simulink model "cst_robotarm1"  (R2020a)
settings: Solver=ode23t  StartTime=0.0  StopTime=5  FixedStep=0.0001  MaxStep=0.05  RelTol=1e-3  EnableMultiTasking=on
model workspace (MAT data in the model file):
  DCMotor_J = 0.0946866703633
  DCMotor_K = 0.477771340295
  DCMotor_Kf = 0.921434142151
  DCMotor_L = 0.000316454712175
  DCMotor_R = 4.99938152603
  Ts = 0.1
  dFilt = [1 -0.1202]
  nFilt = [0.4399 0.4399]
undefined symbols (not defined in the file or in its folder): X, Y, Z
libraries: sm_lib x244, fl_lib x75, nesl_utility x28, ee_lib x21, simulink x6
(part 1 of 6)
settings Model: SimulationMode=accelerator  Creator=The MathWorks, Inc.  LastModifiedBy=nikhil
settings DataIOCC: LimitDataPoints=on  SaveFormat=Array  InspectSignalLogs=on  SaveTime=off  ReturnWorkspaceOutputs=off
settings OptimizationCC: ExpressionDepthLimit=2147483647  LifeSpan=inf
settings DebuggingCC: UnderspecifiedInitializationDetection=Classic  MergeDetectMultiDrivingBlocksExec=none  FcnCallInpInsideContextMsg=warning  StateNameClashWarn=warning  SFUnexpectedBacktrackingDiag=warning  SFNoUnconditionalDefaultTransitionDiag=warning  SFExecutionAtInitializationDiag=none  ArithmeticOperatorsInVariantConditions=warning
settings HardwareCC: ProdBitPerPointer=32  ProdBitPerSizeT=32  ProdBitPerPtrDiffT=32  ProdLargestAtomicFloat=None  ProdIntDivRoundTo=Undefined  ProdEndianess=Unspecified  ProdWordSize=32  ProdHWDeviceType=32-bit Generic
settings ModelReferenceCC: PropagateSignalLabelsOutOfModel=off
settings SFSimCC: SimUseLocalCustomCode=off  CustomCodeUndefinedFunction=UseInterfaceOnly
settings RTWCC: RTWUseLocalCustomCode=off
settings CodeAppCC: StateflowObjectComments=on
settings GRTTargetCC: TargetLangStandard=C89/C90 (ANSI)  CombineOutputUpdateFcns=off  GRTInterface=on
settings ConfigComp: CovMetricSettings=dw  CovHtmlReporting=on  CovSaveCumulativeToWorkspaceVar=on  CovSaveSingleToWorkspaceVar=on  CovExternalEMLEnable=off  CovSFcnEnable=off
settings SimscapeCC: SimscapeNormalizeSystem=off
settings ConfigurationSet: Description=SimMechanics 2G
settings DiagnosticsConfigSet: SimMechanicsUnconnectedFramePorts=none
settings ExplorerConfigSet: SimMechanicsOpenEditorOnUpdate=off  InternalSimMechanicsExplorerSettings="<ExplorerConfiguration><canonicalview>planar_xy</canonicalview><AnimationSetting><BasePlaybackSpeed>1.0</BasePlaybackSpeed><PlaybackSpeedFactor>1.0</PlaybackSpeedFactor></AnimationSetting><TilePanel><TileInfo><Tiles Columns=\"1\" Count=\"1\" Rows=\"1\"><Column Left=\"2\" Weight=\"1\"/><Column Left=\"708\"/><Row Top=\"2\" Weight=\"1\"/><Row Top=\"595\"/><Tile Height=\"1\" Width=\"1\" X=\"0\" Y=\"0\"/></Tiles></TileInfo><SceneInfo><SceneViewer><BGColor><R>0.80000001192092896</R><G>0.80000001192092896</G><B>0.80000001192092896</B></BGColor><Camera><Position><X>0.30752487944302698</X><Y>0.57922836563106395</Y><Z>0.35651305744246536</Z></Position><Center><X>-0.033772386749033274</X><Y>0.23793109943898419</Y><Z>0.015215791250393121</Z></Center><Up><X>-0.40824829046386307</X><Y>0.81649658092772615</Y><Z>-0.40824829046386307</Z></Up><Left>-0.063283674940751766</Left><Right>0.063283674940751766</Right><Bottom>-0.22321517040744418</Bottom><Top>0.22321517040744418</Top></Camera></SceneViewer></SceneInfo></TilePanel></ExplorerConfiguration>"

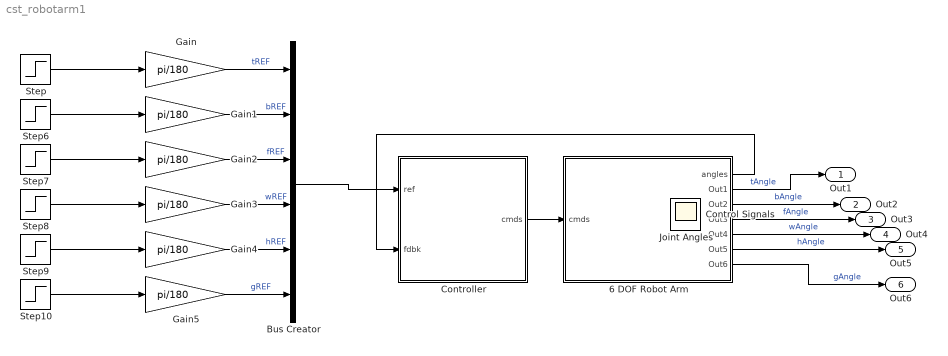
== system cst_robotarm1 ==
  6 DOF Robot Arm : Subsystem
      mask Display: image('RobotArmSystem.jpg',[0.2 0.05 0.6 0.9])
  Bus Creator : BusCreator  Inputs=6
  Controller : Subsystem
  Gain{,1..5} (6 alike) : Gain  Gain=pi/180
  Step : Step  Time=0  After=60  SampleTime=Ts
  Step10 : Step  Time=0  After=60  SampleTime=Ts
  Step6 : Step  Time=0  Before=90  After=80  SampleTime=Ts
  Step7 : Step  Time=0  After=60  SampleTime=Ts
  Step8 : Step  Time=0  After=90  SampleTime=Ts
  Step9 : Step  Time=0  After=90  SampleTime=Ts
  Out1 : Outport
  Out2 : Outport  Port=2
  Out3 : Outport  Port=3
  Out4 : Outport  Port=4
  Out5 : Outport  Port=5
  Out6 : Outport  Port=6
  Control Signals : Scope
  Joint Angles : Scope
  wires:
  Controller/1(cmds) -> 6 DOF Robot Arm/1(cmds)
  6 DOF Robot Arm/1(angles) -> Controller/2(fdbk)
  Gain4/1 -> Bus Creator/5  "hREF"
  Gain/1 -> Bus Creator/1  "tREF"
  Gain3/1 -> Bus Creator/4  "wREF"
  Gain5/1 -> Bus Creator/6  "gREF"
  Gain1/1 -> Bus Creator/2  "bREF"
  Step9/1 -> Gain4/1
  Step/1 -> Gain/1
  Step10/1 -> Gain5/1
  Bus Creator/1 -> Controller/1(ref)
  Gain2/1 -> Bus Creator/3  "fREF"
  Step7/1 -> Gain2/1
  Step8/1 -> Gain3/1
  Step6/1 -> Gain1/1
  6 DOF Robot Arm/2(Out1) -> Out1/1  "tAngle"
  6 DOF Robot Arm/3(Out2) -> Out2/1  "bAngle"
  6 DOF Robot Arm/4(Out3) -> Out3/1  "fAngle"
  6 DOF Robot Arm/5(Out4) -> Out4/1  "wAngle"
  6 DOF Robot Arm/6(Out5) -> Out5/1  "hAngle"
  6 DOF Robot Arm/7(Out6) -> Out6/1  "gAngle"

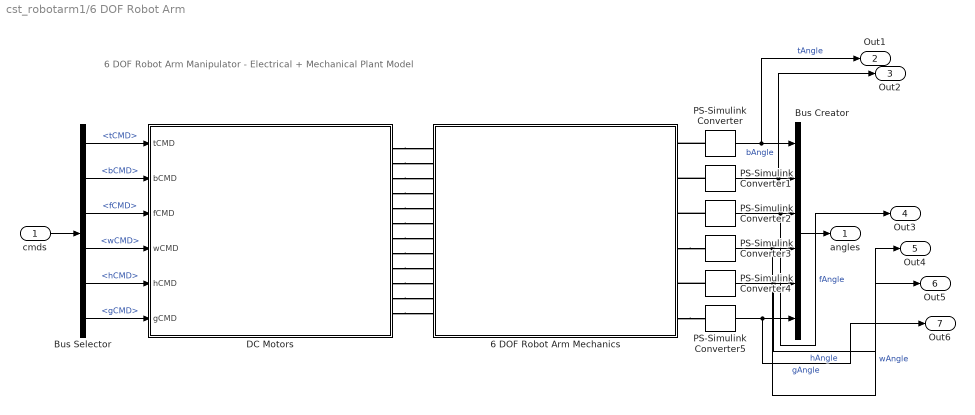
== system cst_robotarm1/6 DOF Robot Arm ==
  note: 6 DOF Robot Arm Manipulator - Electrical + Mechanical Plant Model
  cmds : Inport
  6 DOF Robot Arm Mechanics : Subsystem
      mask Display: image('RobotArm_Mechanics.jpg',[0.1 0 0.8 1])
  Bus Creator : BusCreator  Inputs=6
  Bus Selector : BusSelector  OutputSignals=tCMD,bCMD,fCMD,wCMD,hCMD,gCMD
  DC Motors : Subsystem
      mask Display: image('MultiServos.jpg',[0.25 0.1 0.5 0.8])
  PS-Simulink Converter{,1..5} (6 alike) : nesl_utility/PS-Simulink Converter  PhysicalDomain=network_engine_domain  SubClassName=ps_output  LeftPortType=input  RightPortType=output  PseudoPeriodic=off  Frequencies=[]  Unit=rad  AffineConversion=off
      settings: SourceProductBaseCode=MT,SS
  angles : Outport  VectorParamsAs1DForOutWhenUnconnected=off
  Out1 : Outport  Port=2
  Out2 : Outport  Port=3
  Out3 : Outport  Port=4
  Out4 : Outport  Port=5
  Out5 : Outport  Port=6
  Out6 : Outport  Port=7
  wires:
  Bus Creator/1 -> angles/1
  PS-Simulink Converter2/1 -> Out3/1, Bus Creator/3  "fAngle"
  PS-Simulink Converter5/1 -> Out6/1, Bus Creator/6  "gAngle"
  PS-Simulink Converter/1 -> Out1/1, Bus Creator/1  "tAngle"
  PS-Simulink Converter1/1 -> Out2/1, Bus Creator/2  "bAngle"
  PS-Simulink Converter3/1 -> Out4/1, Bus Creator/4  "wAngle"
  PS-Simulink Converter4/1 -> Out5/1, Bus Creator/5  "hAngle"
  Bus Selector/6 -> DC Motors/6(gCMD)  "<gCMD>"
  Bus Selector/3 -> DC Motors/3(fCMD)  "<fCMD>"
  Bus Selector/4 -> DC Motors/4(wCMD)  "<wCMD>"
  Bus Selector/2 -> DC Motors/2(bCMD)  "<bCMD>"
  Bus Selector/5 -> DC Motors/5(hCMD)  "<hCMD>"
  Bus Selector/1 -> DC Motors/1(tCMD)  "<tCMD>"
  cmds/1 -> Bus Selector/1
  connections:
  PS-Simulink Converter2/LConn1 -- 6 DOF Robot Arm Mechanics/RConn3
  DC Motors/RConn7 -- 6 DOF Robot Arm Mechanics/LConn7
  DC Motors/RConn8 -- 6 DOF Robot Arm Mechanics/LConn8
  DC Motors/RConn6 -- 6 DOF Robot Arm Mechanics/LConn6
  PS-Simulink Converter/LConn1 -- 6 DOF Robot Arm Mechanics/RConn1
  DC Motors/RConn2 -- 6 DOF Robot Arm Mechanics/LConn2
  DC Motors/RConn5 -- 6 DOF Robot Arm Mechanics/LConn5
  DC Motors/RConn11 -- 6 DOF Robot Arm Mechanics/LConn11
  DC Motors/RConn12 -- 6 DOF Robot Arm Mechanics/LConn12
  DC Motors/RConn9 -- 6 DOF Robot Arm Mechanics/LConn9
  DC Motors/RConn3 -- 6 DOF Robot Arm Mechanics/LConn3
  DC Motors/RConn4 -- 6 DOF Robot Arm Mechanics/LConn4
  PS-Simulink Converter1/LConn1 -- 6 DOF Robot Arm Mechanics/RConn2
  PS-Simulink Converter4/LConn1 -- 6 DOF Robot Arm Mechanics/RConn5
  6 DOF Robot Arm Mechanics/RConn6 -- PS-Simulink Converter5/LConn1
  6 DOF Robot Arm Mechanics/RConn4 -- PS-Simulink Converter3/LConn1
  DC Motors/RConn10 -- 6 DOF Robot Arm Mechanics/LConn10
  DC Motors/RConn1 -- 6 DOF Robot Arm Mechanics/LConn1

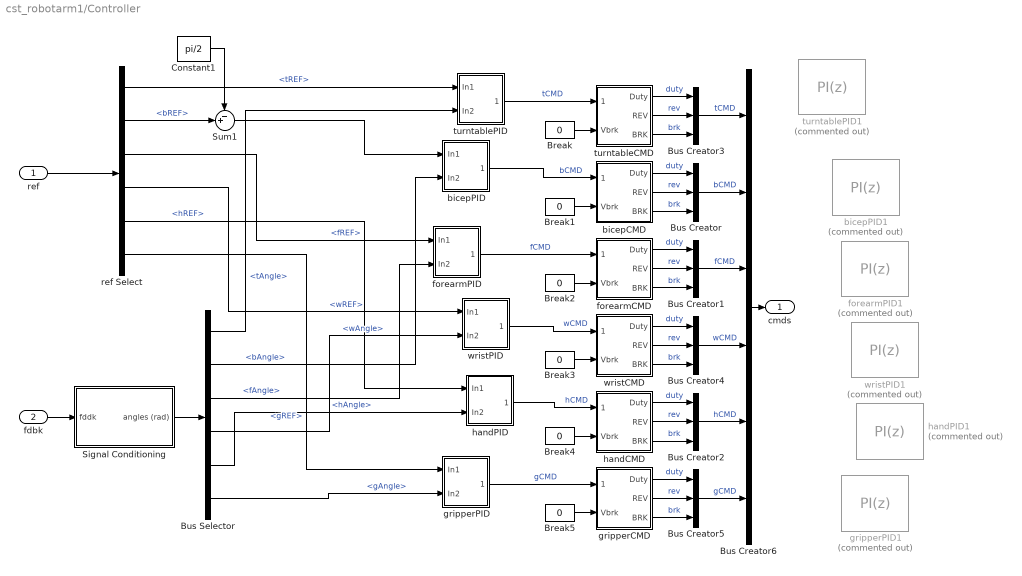
== system cst_robotarm1/Controller ==
  ref : Inport
  fdbk : Inport  Port=2
  Break{,1..5} (6 alike) : Constant  Value=0
  Bus Creator{,1..5} (6 alike) : BusCreator  Inputs=3
  Bus Creator6 : BusCreator  Inputs=6
  Bus Selector : BusSelector  OutputSignals=tAngle,bAngle,fAngle,wAngle,hAngle,gAngle
  Constant1 : Constant  Value=pi/2
  Signal Conditioning : Subsystem
  Sum1 : Sum  Inputs=-+|
  bicepCMD : Subsystem
  bicepPID : Subsystem
  bicepPID1 : simulink/Continuous/PID Controller (2DOF)  Commented=on  Controller=PI  Form=Parallel  TimeDomain=Discrete-time  UseExternalTs=off  SampleTime=Ts  IntegratorMethod=Forward Euler  FilterMethod=Backward Euler  ControllerParametersSource=internal  P=17.4067710058822  I=19.2817621248792  D=2.0  UseFilter=on  N=25  b=1  c=1  TunerSelectOption=Transfer Function Based (PID Tuner App)  InitialConditionSource=internal  InitialConditionForIntegrator=0  InitialConditionForFilter=0  DifferentiatorICPrevScaledInput=0  ExternalReset=none  TrackingMode=off  Kt=1  LimitOutput=on  UpperSaturationLimit=5  LowerSaturationLimit=-5  LinearizeAsGain=on  AntiWindupMode=clamping  Kb=1  POutMin=[]  POutMax=[]  IOutMin=[]  IOutMax=[]  DOutMin=[]  DOutMax=[]  NOutMin=[]  NOutMax=[]  bOutMin=[]  bOutMax=[]  cOutMin=[]  cOutMax=[]  SumOutMin=[]  SumOutMax=[]  SaturationOutMin=[]  SaturationOutMax=[]  PParamMin=[]  PParamMax=[]  IParamMin=[]  IParamMax=[]  DParamMin=[]  DParamMax=[]  NParamMin=[]  NParamMax=[]  bParamMin=[]  bParamMax=[]  cParamMin=[]  cParamMax=[]  KbParamMin=[]  KbParamMax=[]  KtParamMin=[]  KtParamMax=[]  KbOutMin=[]  KbOutMax=[]  KtOutMin=[]  KtOutMax=[]  IntegratorOutMin=[]  IntegratorOutMax=[]  FilterOutMin=[]  FilterOutMax=[]  SumI1OutMin=[]  SumI1OutMax=[]  SumI2OutMin=[]  SumI2OutMax=[]  SumI3OutMin=[]  SumI3OutMax=[]  SumI4OutMin=[]  SumI4OutMax=[]  SumDOutMin=[]  SumDOutMax=[]  Sum1OutMin=[]  Sum1OutMax=[]  Sum2OutMin=[]  Sum2OutMax=[]  Sum3OutMin=[]  Sum3OutMax=[]  DifferentiatorOutMin=[]  DifferentiatorOutMax=[]  FilterDiffOutCoefMin=[]  FilterDiffOutCoefMax=[]  ReciprocalOutMin=[]  ReciprocalOutMax=[]  SumDenOutMin=[]  SumDenOutMax=[]  SumNumOutMin=[]  SumNumOutMax=[]  DivideOutMin=[]  DivideOutMax=[]  UdiffTsProdOutMin=[]  UdiffTsProdOutMax=[]  NTsProdOutMin=[]  NTsProdOutMax=[]  UintegralTsProdOutMin=[]  UintegralTsProdOutMax=[]  UngainTsProdOutMin=[]  UngainTsProdOutMax=[]  IntegratorContinuousStateAttributes=''  IntegratorStateMustResolveToSignalObject=off  IntegratorRTWStateStorageClass=Auto  FilterContinuousStateAttributes=''  FilterStateMustResolveToSignalObject=off  FilterRTWStateStorageClass=Auto  ParallelPVariant=InternalParameters  IdealPVariant=Disabled  IVariant=InternalParameters  DVariant=Disabled  bVariant=InternalParameters  cVariant=Disabled  IntegratorVariant=Discrete  SatVariant=Enabled  AWVariant=DiscClampingParallel  PCopyVariant=Disabled  TRVariant=Disabled  FdbkBlocksVariant=Forward  IdealPFdbkVariant=Disabled  SatFdbkVariant=Disabled  DerivativeFilterVariant=Disabled  NVariant=Disabled  NCopyVariant=Disabled_SignalSpec  FilterICVariant=Disabled  IntegratorICVariant=InternalICs  ExternalResetVariant=Disabled  TRSumVariant=Passthrough  SumFdbkVariant=Disabled  SumVariant=Sum_PI  TsampFilterVariant=InternalTs  TsampNgainVariant=Passthrough  TsampIntegralVariant=Passthrough
  forearmCMD : Subsystem
  forearmPID : Subsystem
  forearmPID1 : simulink/Continuous/PID Controller (2DOF)  Commented=on  Controller=PI  Form=Parallel  TimeDomain=Discrete-time  UseExternalTs=off  SampleTime=Ts  IntegratorMethod=Forward Euler  FilterMethod=Backward Euler  ControllerParametersSource=internal  P=12.4040077539239  I=11.6911006016264  D=2.0  UseFilter=on  N=25  b=1  c=1  TunerSelectOption=Transfer Function Based (PID Tuner App)  InitialConditionSource=internal  InitialConditionForIntegrator=0  InitialConditionForFilter=0  DifferentiatorICPrevScaledInput=0  ExternalReset=none  TrackingMode=off  Kt=1  LimitOutput=on  UpperSaturationLimit=5  LowerSaturationLimit=-5  LinearizeAsGain=on  AntiWindupMode=clamping  Kb=1  POutMin=[]  POutMax=[]  IOutMin=[]  IOutMax=[]  DOutMin=[]  DOutMax=[]  NOutMin=[]  NOutMax=[]  bOutMin=[]  bOutMax=[]  cOutMin=[]  cOutMax=[]  SumOutMin=[]  SumOutMax=[]  SaturationOutMin=[]  SaturationOutMax=[]  PParamMin=[]  PParamMax=[]  IParamMin=[]  IParamMax=[]  DParamMin=[]  DParamMax=[]  NParamMin=[]  NParamMax=[]  bParamMin=[]  bParamMax=[]  cParamMin=[]  cParamMax=[]  KbParamMin=[]  KbParamMax=[]  KtParamMin=[]  KtParamMax=[]  KbOutMin=[]  KbOutMax=[]  KtOutMin=[]  KtOutMax=[]  IntegratorOutMin=[]  IntegratorOutMax=[]  FilterOutMin=[]  FilterOutMax=[]  SumI1OutMin=[]  SumI1OutMax=[]  SumI2OutMin=[]  SumI2OutMax=[]  SumI3OutMin=[]  SumI3OutMax=[]  SumI4OutMin=[]  SumI4OutMax=[]  SumDOutMin=[]  SumDOutMax=[]  Sum1OutMin=[]  Sum1OutMax=[]  Sum2OutMin=[]  Sum2OutMax=[]  Sum3OutMin=[]  Sum3OutMax=[]  DifferentiatorOutMin=[]  DifferentiatorOutMax=[]  FilterDiffOutCoefMin=[]  FilterDiffOutCoefMax=[]  ReciprocalOutMin=[]  ReciprocalOutMax=[]  SumDenOutMin=[]  SumDenOutMax=[]  SumNumOutMin=[]  SumNumOutMax=[]  DivideOutMin=[]  DivideOutMax=[]  UdiffTsProdOutMin=[]  UdiffTsProdOutMax=[]  NTsProdOutMin=[]  NTsProdOutMax=[]  UintegralTsProdOutMin=[]  UintegralTsProdOutMax=[]  UngainTsProdOutMin=[]  UngainTsProdOutMax=[]  IntegratorContinuousStateAttributes=''  IntegratorStateMustResolveToSignalObject=off  IntegratorRTWStateStorageClass=Auto  FilterContinuousStateAttributes=''  FilterStateMustResolveToSignalObject=off  FilterRTWStateStorageClass=Auto  ParallelPVariant=InternalParameters  IdealPVariant=Disabled  IVariant=InternalParameters  DVariant=Disabled  bVariant=InternalParameters  cVariant=Disabled  IntegratorVariant=Discrete  SatVariant=Enabled  AWVariant=DiscClampingParallel  PCopyVariant=Disabled  TRVariant=Disabled  FdbkBlocksVariant=Forward  IdealPFdbkVariant=Disabled  SatFdbkVariant=Disabled  DerivativeFilterVariant=Disabled  NVariant=Disabled  NCopyVariant=Disabled_SignalSpec  FilterICVariant=Disabled  IntegratorICVariant=InternalICs  ExternalResetVariant=Disabled  TRSumVariant=Passthrough  SumFdbkVariant=Disabled  SumVariant=Sum_PI  TsampFilterVariant=InternalTs  TsampNgainVariant=Passthrough  TsampIntegralVariant=Passthrough
  gripperCMD : Subsystem
  gripperPID : Subsystem
  gripperPID1 : simulink/Continuous/PID Controller (2DOF)  Commented=on  Controller=PI  Form=Parallel  TimeDomain=Discrete-time  UseExternalTs=off  SampleTime=Ts  IntegratorMethod=Forward Euler  FilterMethod=Backward Euler  ControllerParametersSource=internal  P=12.0690613111296  I=10.8431971341097  D=2.0  UseFilter=on  N=25  b=1  c=1  TunerSelectOption=Transfer Function Based (PID Tuner App)  InitialConditionSource=internal  InitialConditionForIntegrator=0  InitialConditionForFilter=0  DifferentiatorICPrevScaledInput=0  ExternalReset=none  TrackingMode=off  Kt=1  LimitOutput=on  UpperSaturationLimit=5  LowerSaturationLimit=-5  LinearizeAsGain=on  AntiWindupMode=clamping  Kb=1  POutMin=[]  POutMax=[]  IOutMin=[]  IOutMax=[]  DOutMin=[]  DOutMax=[]  NOutMin=[]  NOutMax=[]  bOutMin=[]  bOutMax=[]  cOutMin=[]  cOutMax=[]  SumOutMin=[]  SumOutMax=[]  SaturationOutMin=[]  SaturationOutMax=[]  PParamMin=[]  PParamMax=[]  IParamMin=[]  IParamMax=[]  DParamMin=[]  DParamMax=[]  NParamMin=[]  NParamMax=[]  bParamMin=[]  bParamMax=[]  cParamMin=[]  cParamMax=[]  KbParamMin=[]  KbParamMax=[]  KtParamMin=[]  KtParamMax=[]  KbOutMin=[]  KbOutMax=[]  KtOutMin=[]  KtOutMax=[]  IntegratorOutMin=[]  IntegratorOutMax=[]  FilterOutMin=[]  FilterOutMax=[]  SumI1OutMin=[]  SumI1OutMax=[]  SumI2OutMin=[]  SumI2OutMax=[]  SumI3OutMin=[]  SumI3OutMax=[]  SumI4OutMin=[]  SumI4OutMax=[]  SumDOutMin=[]  SumDOutMax=[]  Sum1OutMin=[]  Sum1OutMax=[]  Sum2OutMin=[]  Sum2OutMax=[]  Sum3OutMin=[]  Sum3OutMax=[]  DifferentiatorOutMin=[]  DifferentiatorOutMax=[]  FilterDiffOutCoefMin=[]  FilterDiffOutCoefMax=[]  ReciprocalOutMin=[]  ReciprocalOutMax=[]  SumDenOutMin=[]  SumDenOutMax=[]  SumNumOutMin=[]  SumNumOutMax=[]  DivideOutMin=[]  DivideOutMax=[]  UdiffTsProdOutMin=[]  UdiffTsProdOutMax=[]  NTsProdOutMin=[]  NTsProdOutMax=[]  UintegralTsProdOutMin=[]  UintegralTsProdOutMax=[]  UngainTsProdOutMin=[]  UngainTsProdOutMax=[]  IntegratorContinuousStateAttributes=''  IntegratorStateMustResolveToSignalObject=off  IntegratorRTWStateStorageClass=Auto  FilterContinuousStateAttributes=''  FilterStateMustResolveToSignalObject=off  FilterRTWStateStorageClass=Auto  ParallelPVariant=InternalParameters  IdealPVariant=Disabled  IVariant=InternalParameters  DVariant=Disabled  bVariant=InternalParameters  cVariant=Disabled  IntegratorVariant=Discrete  SatVariant=Enabled  AWVariant=DiscClampingParallel  PCopyVariant=Disabled  TRVariant=Disabled  FdbkBlocksVariant=Forward  IdealPFdbkVariant=Disabled  SatFdbkVariant=Disabled  DerivativeFilterVariant=Disabled  NVariant=Disabled  NCopyVariant=Disabled_SignalSpec  FilterICVariant=Disabled  IntegratorICVariant=InternalICs  ExternalResetVariant=Disabled  TRSumVariant=Passthrough  SumFdbkVariant=Disabled  SumVariant=Sum_PI  TsampFilterVariant=InternalTs  TsampNgainVariant=Passthrough  TsampIntegralVariant=Passthrough
  handCMD : Subsystem
  handPID : Subsystem
  handPID1 : simulink/Continuous/PID Controller (2DOF)  Commented=on  Controller=PI  Form=Parallel  TimeDomain=Discrete-time  UseExternalTs=off  SampleTime=Ts  IntegratorMethod=Forward Euler  FilterMethod=Backward Euler  ControllerParametersSource=internal  P=12.2708071891231  I=11.1809254587796  D=2.0  UseFilter=on  N=25  b=1  c=1  TunerSelectOption=Transfer Function Based (PID Tuner App)  InitialConditionSource=internal  InitialConditionForIntegrator=0  InitialConditionForFilter=0  DifferentiatorICPrevScaledInput=0  ExternalReset=none  TrackingMode=off  Kt=1  LimitOutput=on  UpperSaturationLimit=5  LowerSaturationLimit=-5  LinearizeAsGain=on  AntiWindupMode=clamping  Kb=1  POutMin=[]  POutMax=[]  IOutMin=[]  IOutMax=[]  DOutMin=[]  DOutMax=[]  NOutMin=[]  NOutMax=[]  bOutMin=[]  bOutMax=[]  cOutMin=[]  cOutMax=[]  SumOutMin=[]  SumOutMax=[]  SaturationOutMin=[]  SaturationOutMax=[]  PParamMin=[]  PParamMax=[]  IParamMin=[]  IParamMax=[]  DParamMin=[]  DParamMax=[]  NParamMin=[]  NParamMax=[]  bParamMin=[]  bParamMax=[]  cParamMin=[]  cParamMax=[]  KbParamMin=[]  KbParamMax=[]  KtParamMin=[]  KtParamMax=[]  KbOutMin=[]  KbOutMax=[]  KtOutMin=[]  KtOutMax=[]  IntegratorOutMin=[]  IntegratorOutMax=[]  FilterOutMin=[]  FilterOutMax=[]  SumI1OutMin=[]  SumI1OutMax=[]  SumI2OutMin=[]  SumI2OutMax=[]  SumI3OutMin=[]  SumI3OutMax=[]  SumI4OutMin=[]  SumI4OutMax=[]  SumDOutMin=[]  SumDOutMax=[]  Sum1OutMin=[]  Sum1OutMax=[]  Sum2OutMin=[]  Sum2OutMax=[]  Sum3OutMin=[]  Sum3OutMax=[]  DifferentiatorOutMin=[]  DifferentiatorOutMax=[]  FilterDiffOutCoefMin=[]  FilterDiffOutCoefMax=[]  ReciprocalOutMin=[]  ReciprocalOutMax=[]  SumDenOutMin=[]  SumDenOutMax=[]  SumNumOutMin=[]  SumNumOutMax=[]  DivideOutMin=[]  DivideOutMax=[]  UdiffTsProdOutMin=[]  UdiffTsProdOutMax=[]  NTsProdOutMin=[]  NTsProdOutMax=[]  UintegralTsProdOutMin=[]  UintegralTsProdOutMax=[]  UngainTsProdOutMin=[]  UngainTsProdOutMax=[]  IntegratorContinuousStateAttributes=''  IntegratorStateMustResolveToSignalObject=off  IntegratorRTWStateStorageClass=Auto  FilterContinuousStateAttributes=''  FilterStateMustResolveToSignalObject=off  FilterRTWStateStorageClass=Auto  ParallelPVariant=InternalParameters  IdealPVariant=Disabled  IVariant=InternalParameters  DVariant=Disabled  bVariant=InternalParameters  cVariant=Disabled  IntegratorVariant=Discrete  SatVariant=Enabled  AWVariant=DiscClampingParallel  PCopyVariant=Disabled  TRVariant=Disabled  FdbkBlocksVariant=Forward  IdealPFdbkVariant=Disabled  SatFdbkVariant=Disabled  DerivativeFilterVariant=Disabled  NVariant=Disabled  NCopyVariant=Disabled_SignalSpec  FilterICVariant=Disabled  IntegratorICVariant=InternalICs  ExternalResetVariant=Disabled  TRSumVariant=Passthrough  SumFdbkVariant=Disabled  SumVariant=Sum_PI  TsampFilterVariant=InternalTs  TsampNgainVariant=Passthrough  TsampIntegralVariant=Passthrough
  ref Select : BusSelector  OutputSignals=tREF,bREF,fREF,wREF,hREF,gREF
  turntableCMD : Subsystem
  turntablePID : Subsystem
  turntablePID1 : simulink/Continuous/PID Controller (2DOF)  Commented=on  Controller=PI  Form=Parallel  TimeDomain=Discrete-time  UseExternalTs=off  SampleTime=Ts  IntegratorMethod=Forward Euler  FilterMethod=Backward Euler  ControllerParametersSource=internal  P=11.7676137148845  I=10.1997672914671  D=2.0  UseFilter=on  N=25  b=1  c=1  TunerSelectOption=Transfer Function Based (PID Tuner App)  InitialConditionSource=internal  InitialConditionForIntegrator=0  InitialConditionForFilter=0  DifferentiatorICPrevScaledInput=0  ExternalReset=none  TrackingMode=off  Kt=1  LimitOutput=on  UpperSaturationLimit=5  LowerSaturationLimit=-5  LinearizeAsGain=on  AntiWindupMode=clamping  Kb=1  POutMin=[]  POutMax=[]  IOutMin=[]  IOutMax=[]  DOutMin=[]  DOutMax=[]  NOutMin=[]  NOutMax=[]  bOutMin=[]  bOutMax=[]  cOutMin=[]  cOutMax=[]  SumOutMin=[]  SumOutMax=[]  SaturationOutMin=[]  SaturationOutMax=[]  PParamMin=[]  PParamMax=[]  IParamMin=[]  IParamMax=[]  DParamMin=[]  DParamMax=[]  NParamMin=[]  NParamMax=[]  bParamMin=[]  bParamMax=[]  cParamMin=[]  cParamMax=[]  KbParamMin=[]  KbParamMax=[]  KtParamMin=[]  KtParamMax=[]  KbOutMin=[]  KbOutMax=[]  KtOutMin=[]  KtOutMax=[]  IntegratorOutMin=[]  IntegratorOutMax=[]  FilterOutMin=[]  FilterOutMax=[]  SumI1OutMin=[]  SumI1OutMax=[]  SumI2OutMin=[]  SumI2OutMax=[]  SumI3OutMin=[]  SumI3OutMax=[]  SumI4OutMin=[]  SumI4OutMax=[]  SumDOutMin=[]  SumDOutMax=[]  Sum1OutMin=[]  Sum1OutMax=[]  Sum2OutMin=[]  Sum2OutMax=[]  Sum3OutMin=[]  Sum3OutMax=[]  DifferentiatorOutMin=[]  DifferentiatorOutMax=[]  FilterDiffOutCoefMin=[]  FilterDiffOutCoefMax=[]  ReciprocalOutMin=[]  ReciprocalOutMax=[]  SumDenOutMin=[]  SumDenOutMax=[]  SumNumOutMin=[]  SumNumOutMax=[]  DivideOutMin=[]  DivideOutMax=[]  UdiffTsProdOutMin=[]  UdiffTsProdOutMax=[]  NTsProdOutMin=[]  NTsProdOutMax=[]  UintegralTsProdOutMin=[]  UintegralTsProdOutMax=[]  UngainTsProdOutMin=[]  UngainTsProdOutMax=[]  IntegratorContinuousStateAttributes=''  IntegratorStateMustResolveToSignalObject=off  IntegratorRTWStateStorageClass=Auto  FilterContinuousStateAttributes=''  FilterStateMustResolveToSignalObject=off  FilterRTWStateStorageClass=Auto  ParallelPVariant=InternalParameters  IdealPVariant=Disabled  IVariant=InternalParameters  DVariant=Disabled  bVariant=InternalParameters  cVariant=Disabled  IntegratorVariant=Discrete  SatVariant=Enabled  AWVariant=DiscClampingParallel  PCopyVariant=Disabled  TRVariant=Disabled  FdbkBlocksVariant=Forward  IdealPFdbkVariant=Disabled  SatFdbkVariant=Disabled  DerivativeFilterVariant=Disabled  NVariant=Disabled  NCopyVariant=Disabled_SignalSpec  FilterICVariant=Disabled  IntegratorICVariant=InternalICs  ExternalResetVariant=Disabled  TRSumVariant=Passthrough  SumFdbkVariant=Disabled  SumVariant=Sum_PI  TsampFilterVariant=InternalTs  TsampNgainVariant=Passthrough  TsampIntegralVariant=Passthrough
  wristCMD : Subsystem
  wristPID : Subsystem
  wristPID1 : simulink/Continuous/PID Controller (2DOF)  Commented=on  Controller=PI  Form=Parallel  TimeDomain=Discrete-time  UseExternalTs=off  SampleTime=Ts  IntegratorMethod=Forward Euler  FilterMethod=Backward Euler  ControllerParametersSource=internal  P=11.0944145049934  I=9.18313614467805  D=2.0  UseFilter=on  N=25  b=1  c=1  TunerSelectOption=Transfer Function Based (PID Tuner App)  InitialConditionSource=internal  InitialConditionForIntegrator=0  InitialConditionForFilter=0  DifferentiatorICPrevScaledInput=0  ExternalReset=none  TrackingMode=off  Kt=1  LimitOutput=on  UpperSaturationLimit=5  LowerSaturationLimit=-5  LinearizeAsGain=on  AntiWindupMode=clamping  Kb=1  POutMin=[]  POutMax=[]  IOutMin=[]  IOutMax=[]  DOutMin=[]  DOutMax=[]  NOutMin=[]  NOutMax=[]  bOutMin=[]  bOutMax=[]  cOutMin=[]  cOutMax=[]  SumOutMin=[]  SumOutMax=[]  SaturationOutMin=[]  SaturationOutMax=[]  PParamMin=[]  PParamMax=[]  IParamMin=[]  IParamMax=[]  DParamMin=[]  DParamMax=[]  NParamMin=[]  NParamMax=[]  bParamMin=[]  bParamMax=[]  cParamMin=[]  cParamMax=[]  KbParamMin=[]  KbParamMax=[]  KtParamMin=[]  KtParamMax=[]  KbOutMin=[]  KbOutMax=[]  KtOutMin=[]  KtOutMax=[]  IntegratorOutMin=[]  IntegratorOutMax=[]  FilterOutMin=[]  FilterOutMax=[]  SumI1OutMin=[]  SumI1OutMax=[]  SumI2OutMin=[]  SumI2OutMax=[]  SumI3OutMin=[]  SumI3OutMax=[]  SumI4OutMin=[]  SumI4OutMax=[]  SumDOutMin=[]  SumDOutMax=[]  Sum1OutMin=[]  Sum1OutMax=[]  Sum2OutMin=[]  Sum2OutMax=[]  Sum3OutMin=[]  Sum3OutMax=[]  DifferentiatorOutMin=[]  DifferentiatorOutMax=[]  FilterDiffOutCoefMin=[]  FilterDiffOutCoefMax=[]  ReciprocalOutMin=[]  ReciprocalOutMax=[]  SumDenOutMin=[]  SumDenOutMax=[]  SumNumOutMin=[]  SumNumOutMax=[]  DivideOutMin=[]  DivideOutMax=[]  UdiffTsProdOutMin=[]  UdiffTsProdOutMax=[]  NTsProdOutMin=[]  NTsProdOutMax=[]  UintegralTsProdOutMin=[]  UintegralTsProdOutMax=[]  UngainTsProdOutMin=[]  UngainTsProdOutMax=[]  IntegratorContinuousStateAttributes=''  IntegratorStateMustResolveToSignalObject=off  IntegratorRTWStateStorageClass=Auto  FilterContinuousStateAttributes=''  FilterStateMustResolveToSignalObject=off  FilterRTWStateStorageClass=Auto  ParallelPVariant=InternalParameters  IdealPVariant=Disabled  IVariant=InternalParameters  DVariant=Disabled  bVariant=InternalParameters  cVariant=Disabled  IntegratorVariant=Discrete  SatVariant=Enabled  AWVariant=DiscClampingParallel  PCopyVariant=Disabled  TRVariant=Disabled  FdbkBlocksVariant=Forward  IdealPFdbkVariant=Disabled  SatFdbkVariant=Disabled  DerivativeFilterVariant=Disabled  NVariant=Disabled  NCopyVariant=Disabled_SignalSpec  FilterICVariant=Disabled  IntegratorICVariant=InternalICs  ExternalResetVariant=Disabled  TRSumVariant=Passthrough  SumFdbkVariant=Disabled  SumVariant=Sum_PI  TsampFilterVariant=InternalTs  TsampNgainVariant=Passthrough  TsampIntegralVariant=Passthrough
  cmds : Outport  VectorParamsAs1DForOutWhenUnconnected=off
  wires:
  bicepCMD/1(Duty) -> Bus Creator/1  "duty"
  bicepCMD/2(REV) -> Bus Creator/2  "rev"
  bicepCMD/3(BRK) -> Bus Creator/3  "brk"
  forearmCMD/1(Duty) -> Bus Creator1/1  "duty"
  forearmCMD/2(REV) -> Bus Creator1/2  "rev"
  forearmCMD/3(BRK) -> Bus Creator1/3  "brk"
  handCMD/2(REV) -> Bus Creator2/2  "rev"
  handCMD/3(BRK) -> Bus Creator2/3  "brk"
  handCMD/1(Duty) -> Bus Creator2/1  "duty"
  bicepPID/1(Vcmd) -> bicepCMD/1(Vcmd)  "bCMD"
  Break1/1 -> bicepCMD/2(Vbrk)
  forearmPID/1(Vcmd) -> forearmCMD/1(Vcmd)  "fCMD"
  Break2/1 -> forearmCMD/2(Vbrk)
  handPID/1(Vcmd) -> handCMD/1(Vcmd)  "hCMD"
  Break4/1 -> handCMD/2(Vbrk)
  Bus Creator1/1 -> Bus Creator6/3  "fCMD"
  Bus Creator2/1 -> Bus Creator6/5  "hCMD"
  ref/1 -> ref Select/1
  turntableCMD/1(Duty) -> Bus Creator3/1  "duty"
  turntableCMD/2(REV) -> Bus Creator3/2  "rev"
  turntableCMD/3(BRK) -> Bus Creator3/3  "brk"
  turntablePID/1(Vcmd) -> turntableCMD/1(Vcmd)  "tCMD"
  Break/1 -> turntableCMD/2(Vbrk)
  Bus Creator3/1 -> Bus Creator6/1  "tCMD"
  wristCMD/2(REV) -> Bus Creator4/2  "rev"
  wristCMD/3(BRK) -> Bus Creator4/3  "brk"
  wristCMD/1(Duty) -> Bus Creator4/1  "duty"
  wristPID/1(Vcmd) -> wristCMD/1(Vcmd)  "wCMD"
  Break3/1 -> wristCMD/2(Vbrk)
  Bus Creator4/1 -> Bus Creator6/4  "wCMD"
  gripperCMD/2(REV) -> Bus Creator5/2  "rev"
  gripperCMD/3(BRK) -> Bus Creator5/3  "brk"
  gripperCMD/1(Duty) -> Bus Creator5/1  "duty"
  gripperPID/1(Vcmd) -> gripperCMD/1(Vcmd)  "gCMD"
  Break5/1 -> gripperCMD/2(Vbrk)
  Bus Creator5/1 -> Bus Creator6/6  "gCMD"
  Bus Creator/1 -> Bus Creator6/2  "bCMD"
  Bus Creator6/1 -> cmds/1
  Bus Selector/6 -> gripperPID/2(In2)  "<gAngle>"
  Bus Selector/5 -> handPID/2(In2)  "<hAngle>"
  Bus Selector/4 -> wristPID/2(In2)  "<wAngle>"
  Bus Selector/3 -> forearmPID/2(In2)  "<fAngle>"
  Bus Selector/1 -> turntablePID/2(In2)  "<tAngle>"
  ref Select/1 -> turntablePID/1(In1)  "<tREF>"
  ref Select/3 -> forearmPID/1(In1)  "<fREF>"
  ref Select/4 -> wristPID/1(In1)  "<wREF>"
  ref Select/5 -> handPID/1(In1)  "<hREF>"
  ref Select/6 -> gripperPID/1(In1)  "<gREF>"
  fdbk/1 -> Signal Conditioning/1(fddk)
  Signal Conditioning/1(angles (rad)) -> Bus Selector/1
  Sum1/1 -> bicepPID/1(In1)
  ref Select/2 -> Sum1/2  "<bREF>"
  Constant1/1 -> Sum1/1
  Bus Selector/2 -> bicepPID/2(In2)  "<bAngle>"

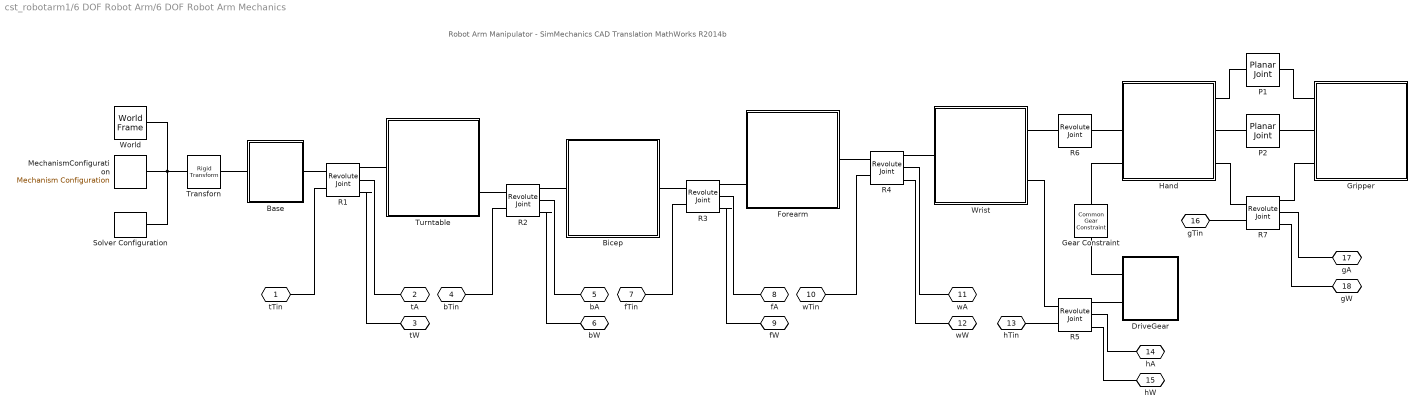
== system cst_robotarm1/6 DOF Robot Arm/6 DOF Robot Arm Mechanics ==
  note: Robot Arm Manipulator - SimMechanics CAD Translation
      | MathWorks R2014b
  Base : Subsystem
      mask Display: image('Base.jpg',[0.25,0.25,0.5,0.5])
  Bicep : Subsystem
      mask Display: image('Bicep.jpg')
  DriveGear : Subsystem
      mask Display: image('DriveGear.jpg',[0.2,0.2,0.6,0.6])
  Forearm : Subsystem
      mask Display: image('Forearm.jpg')
  Gear Constraint : sm_lib/Gears and Couplings/Gears/Common Gear Constraint  GearType=External  SpecificationType=CenterDistanceRatio  CenterDistance=39.8888296  CenterDistanceUnits=mm  GearRatio=1.0  BaseGearRadius=10.0  BaseGearRadiusUnits=cm  FollGearRadius=10.0  FollGearRadiusUnits=cm  AssemblyGearRotation=Free
      settings: SourceProductBaseCode=MS
  Gripper : Subsystem
      mask Display: image('Gripper.jpg',[0.1,0.1,0.8,0.8])
  Hand : Subsystem
      mask Display: image('Hand.jpg',[0.1,0.1,0.8,0.8])
  MechanismConfiguration : sm_lib/Utilities/Mechanism Configuration  UniformGravity=Constant  GravityVector=[0 -9.81 0]  GravityUnits=m/s^2  LinearizationDelta=0.001
  P1 : sm_lib/Joints/Planar Joint  JointMode=Normal  SenseConstraintForce=off  SenseConstraintForceX=off  SenseConstraintForceY=off  SenseConstraintForceZ=off  SenseConstraintTorque=off  SenseConstraintTorqueX=off  SenseConstraintTorqueY=off  SenseConstraintTorqueZ=off  SenseTotalForce=off  SenseTotalForceX=off  SenseTotalForceY=off  SenseTotalForceZ=off  SenseTotalTorque=off  SenseTotalTorqueX=off  SenseTotalTorqueY=off  SenseTotalTorqueZ=off  CompositeWrenchDir=FollowerOnBase  CompositeWrenchFrame=BaseFrame  PxEquilibriumPosition=0  PxEquilibriumPositionUnits=m  PxSpringStiffness=0  PxSpringStiffnessUnits=N/m  PxDampingCoefficient=0  PxDampingCoefficientUnits=s*N/m  PxTorqueActuationMode=NoTorque  PxMotionActuationMode=ComputedMotion  PxSensePosition=off  PxSenseVelocity=off  PxSenseAcceleration=off  PxSenseTorqueForce=off  PxSenseLowerLimitTorqueForce=off  PxSenseUpperLimitTorqueForce=off  PxLowerLimitSpecify=off  PxLowerLimitBound=-1  PxLowerLimitBoundUnits=m  PxLowerLimitStiffness=1e6  PxLowerLimitStiffnessUnits=N/m  PxLowerLimitDamping=1e3  PxLowerLimitDampingUnits=N/(m/s)  PxLowerLimitTransitionRegionWidth=1e-4  PxLowerLimitTransitionRegionWidthUnits=m  PxUpperLimitSpecify=off  PxUpperLimitBound=1  PxUpperLimitBoundUnits=m  PxUpperLimitStiffness=1e6  PxUpperLimitStiffnessUnits=N/m  PxUpperLimitDamping=1e3  PxUpperLimitDampingUnits=N/(m/s)  PxUpperLimitTransitionRegionWidth=1e-4  PxUpperLimitTransitionRegionWidthUnits=m  PxPositionTargetSpecify=off  PxPositionTargetPriority=High  PxPositionTargetValue=0  PxPositionTargetValueUnits=m  PxVelocityTargetSpecify=off  PxVelocityTargetPriority=High  PxVelocityTargetValue=0  PxVelocityTargetValueUnits=m/s  PyEquilibriumPosition=0  PyEquilibriumPositionUnits=m  PySpringStiffness=0  PySpringStiffnessUnits=N/m  PyDampingCoefficient=0  PyDampingCoefficientUnits=s*N/m  PyTorqueActuationMode=NoTorque  PyMotionActuationMode=ComputedMotion  PySensePosition=off  PySenseVelocity=off  PySenseAcceleration=off  PySenseTorqueForce=off  PySenseLowerLimitTorqueForce=off  PySenseUpperLimitTorqueForce=off  PyLowerLimitSpecify=off  PyLowerLimitBound=-1  PyLowerLimitBoundUnits=m  PyLowerLimitStiffness=1e6  PyLowerLimitStiffnessUnits=N/m  PyLowerLimitDamping=1e3  PyLowerLimitDampingUnits=N/(m/s)  PyLowerLimitTransitionRegionWidth=1e-4  PyLowerLimitTransitionRegionWidthUnits=m  PyUpperLimitSpecify=off  PyUpperLimitBound=1  PyUpperLimitBoundUnits=m  PyUpperLimitStiffness=1e6  PyUpperLimitStiffnessUnits=N/m  PyUpperLimitDamping=1e3  PyUpperLimitDampingUnits=N/(m/s)  PyUpperLimitTransitionRegionWidth=1e-4  PyUpperLimitTransitionRegionWidthUnits=m  PyPositionTargetSpecify=off  PyPositionTargetPriority=High  PyPositionTargetValue=0  PyPositionTargetValueUnits=m  PyVelocityTargetSpecify=off  PyVelocityTargetPriority=High  PyVelocityTargetValue=0  PyVelocityTargetValueUnits=m/s  RzEquilibriumPosition=0  RzEquilibriumPositionUnits=rad  RzSpringStiffness=0  RzSpringStiffnessUnits=m*N/rad  RzDampingCoefficient=0  RzDampingCoefficientUnits=m*s*N/rad  RzTorqueActuationMode=NoTorque  RzMotionActuationMode=ComputedMotion  RzSensePosition=off  RzSenseVelocity=off  RzSenseAcceleration=off  RzSenseTorqueForce=off  RzSenseLowerLimitTorqueForce=off  RzSenseUpperLimitTorqueForce=off  RzLowerLimitSpecify=off  RzLowerLimitBound=-90  RzLowerLimitBoundUnits=deg  RzLowerLimitStiffness=1e4  RzLowerLimitStiffnessUnits=N*m/deg  RzLowerLimitDamping=10  RzLowerLimitDampingUnits=N*m/(deg/s)  RzLowerLimitTransitionRegionWidth=0.1  RzLowerLimitTransitionRegionWidthUnits=deg  RzUpperLimitSpecify=off  RzUpperLimitBound=90  RzUpperLimitBoundUnits=deg  RzUpperLimitStiffness=1e4  RzUpperLimitStiffnessUnits=N*m/deg  RzUpperLimitDamping=10  RzUpperLimitDampingUnits=N*m/(deg/s)  RzUpperLimitTransitionRegionWidth=0.1  RzUpperLimitTransitionRegionWidthUnits=deg  RzPositionTargetSpecify=off  RzPositionTargetPriority=High  RzPositionTargetValue=0  RzPositionTargetValueUnits=deg  RzVelocityTargetSpecify=off  RzVelocityTargetPriority=High  RzVelocityTargetValue=0  RzVelocityTargetValueUnits=deg/s
  P2 : sm_lib/Joints/Planar Joint  JointMode=Normal  SenseConstraintForce=off  SenseConstraintForceX=off  SenseConstraintForceY=off  SenseConstraintForceZ=off  SenseConstraintTorque=off  SenseConstraintTorqueX=off  SenseConstraintTorqueY=off  SenseConstraintTorqueZ=off  SenseTotalForce=off  SenseTotalForceX=off  SenseTotalForceY=off  SenseTotalForceZ=off  SenseTotalTorque=off  SenseTotalTorqueX=off  SenseTotalTorqueY=off  SenseTotalTorqueZ=off  CompositeWrenchDir=FollowerOnBase  CompositeWrenchFrame=BaseFrame  PxEquilibriumPosition=0  PxEquilibriumPositionUnits=m  PxSpringStiffness=0  PxSpringStiffnessUnits=N/m  PxDampingCoefficient=0  PxDampingCoefficientUnits=s*N/m  PxTorqueActuationMode=NoTorque  PxMotionActuationMode=ComputedMotion  PxSensePosition=off  PxSenseVelocity=off  PxSenseAcceleration=off  PxSenseTorqueForce=off  PxSenseLowerLimitTorqueForce=off  PxSenseUpperLimitTorqueForce=off  PxLowerLimitSpecify=off  PxLowerLimitBound=-1  PxLowerLimitBoundUnits=m  PxLowerLimitStiffness=1e6  PxLowerLimitStiffnessUnits=N/m  PxLowerLimitDamping=1e3  PxLowerLimitDampingUnits=N/(m/s)  PxLowerLimitTransitionRegionWidth=1e-4  PxLowerLimitTransitionRegionWidthUnits=m  PxUpperLimitSpecify=off  PxUpperLimitBound=1  PxUpperLimitBoundUnits=m  PxUpperLimitStiffness=1e6  PxUpperLimitStiffnessUnits=N/m  PxUpperLimitDamping=1e3  PxUpperLimitDampingUnits=N/(m/s)  PxUpperLimitTransitionRegionWidth=1e-4  PxUpperLimitTransitionRegionWidthUnits=m  PxPositionTargetSpecify=off  PxPositionTargetPriority=High  PxPositionTargetValue=0  PxPositionTargetValueUnits=m  PxVelocityTargetSpecify=off  PxVelocityTargetPriority=High  PxVelocityTargetValue=0  PxVelocityTargetValueUnits=m/s  PyEquilibriumPosition=0  PyEquilibriumPositionUnits=m  PySpringStiffness=0  PySpringStiffnessUnits=N/m  PyDampingCoefficient=0  PyDampingCoefficientUnits=s*N/m  PyTorqueActuationMode=NoTorque  PyMotionActuationMode=ComputedMotion  PySensePosition=off  PySenseVelocity=off  PySenseAcceleration=off  PySenseTorqueForce=off  PySenseLowerLimitTorqueForce=off  PySenseUpperLimitTorqueForce=off  PyLowerLimitSpecify=off  PyLowerLimitBound=-1  PyLowerLimitBoundUnits=m  PyLowerLimitStiffness=1e6  PyLowerLimitStiffnessUnits=N/m  PyLowerLimitDamping=1e3  PyLowerLimitDampingUnits=N/(m/s)  PyLowerLimitTransitionRegionWidth=1e-4  PyLowerLimitTransitionRegionWidthUnits=m  PyUpperLimitSpecify=off  PyUpperLimitBound=1  PyUpperLimitBoundUnits=m  PyUpperLimitStiffness=1e6  PyUpperLimitStiffnessUnits=N/m  PyUpperLimitDamping=1e3  PyUpperLimitDampingUnits=N/(m/s)  PyUpperLimitTransitionRegionWidth=1e-4  PyUpperLimitTransitionRegionWidthUnits=m  PyPositionTargetSpecify=off  PyPositionTargetPriority=High  PyPositionTargetValue=0  PyPositionTargetValueUnits=m  PyVelocityTargetSpecify=off  PyVelocityTargetPriority=High  PyVelocityTargetValue=0  PyVelocityTargetValueUnits=m/s  RzEquilibriumPosition=0  RzEquilibriumPositionUnits=rad  RzSpringStiffness=0  RzSpringStiffnessUnits=m*N/rad  RzDampingCoefficient=0  RzDampingCoefficientUnits=m*s*N/rad  RzTorqueActuationMode=NoTorque  RzMotionActuationMode=ComputedMotion  RzSensePosition=off  RzSenseVelocity=off  RzSenseAcceleration=off  RzSenseTorqueForce=off  RzSenseLowerLimitTorqueForce=off  RzSenseUpperLimitTorqueForce=off  RzLowerLimitSpecify=off  RzLowerLimitBound=-90  RzLowerLimitBoundUnits=deg  RzLowerLimitStiffness=1e4  RzLowerLimitStiffnessUnits=N*m/deg  RzLowerLimitDamping=10  RzLowerLimitDampingUnits=N*m/(deg/s)  RzLowerLimitTransitionRegionWidth=0.1  RzLowerLimitTransitionRegionWidthUnits=deg  RzUpperLimitSpecify=off  RzUpperLimitBound=90  RzUpperLimitBoundUnits=deg  RzUpperLimitStiffness=1e4  RzUpperLimitStiffnessUnits=N*m/deg  RzUpperLimitDamping=10  RzUpperLimitDampingUnits=N*m/(deg/s)  RzUpperLimitTransitionRegionWidth=0.1  RzUpperLimitTransitionRegionWidthUnits=deg  RzPositionTargetSpecify=off  RzPositionTargetPriority=High  RzPositionTargetValue=0  RzPositionTargetValueUnits=deg  RzVelocityTargetSpecify=off  RzVelocityTargetPriority=High  RzVelocityTargetValue=0  RzVelocityTargetValueUnits=deg/s
  R{1,3..5,7} (5 alike) : sm_lib/Joints/Revolute Joint  JointMode=Normal  SenseConstraintForce=off  SenseConstraintForceX=off  SenseConstraintForceY=off  SenseConstraintForceZ=off  SenseConstraintTorque=off  SenseConstraintTorqueX=off  SenseConstraintTorqueY=off  SenseConstraintTorqueZ=off  SenseTotalForce=off  SenseTotalForceX=off  SenseTotalForceY=off  SenseTotalForceZ=off  SenseTotalTorque=off  SenseTotalTorqueX=off  SenseTotalTorqueY=off  SenseTotalTorqueZ=off  CompositeWrenchDir=FollowerOnBase  CompositeWrenchFrame=BaseFrame  EquilibriumPosition=0  EquilibriumPositionUnits=rad  SpringStiffness=0  SpringStiffnessUnits=m*N/rad  DampingCoefficient=0  DampingCoefficientUnits=m*s*N/rad  TorqueActuationMode=InputTorque  MotionActuationMode=ComputedMotion  SensePosition=on  SenseVelocity=on  SenseAcceleration=off  SenseTorqueForce=off  SenseLowerLimitTorqueForce=off  SenseUpperLimitTorqueForce=off  LowerLimitSpecify=off  LowerLimitBound=-90  LowerLimitBoundUnits=deg  LowerLimitStiffness=1e4  LowerLimitStiffnessUnits=N*m/deg  LowerLimitDamping=10  LowerLimitDampingUnits=N*m/(deg/s)  LowerLimitTransitionRegionWidth=0.1  LowerLimitTransitionRegionWidthUnits=deg  UpperLimitSpecify=off  UpperLimitBound=90  UpperLimitBoundUnits=deg  UpperLimitStiffness=1e4  UpperLimitStiffnessUnits=N*m/deg  UpperLimitDamping=10  UpperLimitDampingUnits=N*m/(deg/s)  UpperLimitTransitionRegionWidth=0.1  UpperLimitTransitionRegionWidthUnits=deg  PositionTargetSpecify=on  PositionTargetPriority=High  PositionTargetValue=0  PositionTargetValueUnits=deg  VelocityTargetSpecify=on  VelocityTargetPriority=High  VelocityTargetValue=0  VelocityTargetValueUnits=deg/s
  R2 : sm_lib/Joints/Revolute Joint  JointMode=Normal  SenseConstraintForce=off  SenseConstraintForceX=off  SenseConstraintForceY=off  SenseConstraintForceZ=off  SenseConstraintTorque=off  SenseConstraintTorqueX=off  SenseConstraintTorqueY=off  SenseConstraintTorqueZ=off  SenseTotalForce=off  SenseTotalForceX=off  SenseTotalForceY=off  SenseTotalForceZ=off  SenseTotalTorque=off  SenseTotalTorqueX=off  SenseTotalTorqueY=off  SenseTotalTorqueZ=off  CompositeWrenchDir=FollowerOnBase  CompositeWrenchFrame=BaseFrame  EquilibriumPosition=0  EquilibriumPositionUnits=rad  SpringStiffness=0  SpringStiffnessUnits=m*N/rad  DampingCoefficient=0  DampingCoefficientUnits=m*s*N/rad  TorqueActuationMode=InputTorque  MotionActuationMode=ComputedMotion  SensePosition=on  SenseVelocity=on  SenseAcceleration=off  SenseTorqueForce=off  SenseLowerLimitTorqueForce=off  SenseUpperLimitTorqueForce=off  LowerLimitSpecify=off  LowerLimitBound=-90  LowerLimitBoundUnits=deg  LowerLimitStiffness=1e4  LowerLimitStiffnessUnits=N*m/deg  LowerLimitDamping=10  LowerLimitDampingUnits=N*m/(deg/s)  LowerLimitTransitionRegionWidth=0.1  LowerLimitTransitionRegionWidthUnits=deg  UpperLimitSpecify=off  UpperLimitBound=90  UpperLimitBoundUnits=deg  UpperLimitStiffness=1e4  UpperLimitStiffnessUnits=N*m/deg  UpperLimitDamping=10  UpperLimitDampingUnits=N*m/(deg/s)  UpperLimitTransitionRegionWidth=0.1  UpperLimitTransitionRegionWidthUnits=deg  PositionTargetSpecify=on  PositionTargetPriority=High  PositionTargetValue=90  PositionTargetValueUnits=deg  VelocityTargetSpecify=on  VelocityTargetPriority=High  VelocityTargetValue=0  VelocityTargetValueUnits=deg/s
  R6 : sm_lib/Joints/Revolute Joint  JointMode=Normal  SenseConstraintForce=off  SenseConstraintForceX=off  SenseConstraintForceY=off  SenseConstraintForceZ=off  SenseConstraintTorque=off  SenseConstraintTorqueX=off  SenseConstraintTorqueY=off  SenseConstraintTorqueZ=off  SenseTotalForce=off  SenseTotalForceX=off  SenseTotalForceY=off  SenseTotalForceZ=off  SenseTotalTorque=off  SenseTotalTorqueX=off  SenseTotalTorqueY=off  SenseTotalTorqueZ=off  CompositeWrenchDir=FollowerOnBase  CompositeWrenchFrame=BaseFrame  EquilibriumPosition=0  EquilibriumPositionUnits=rad  SpringStiffness=0  SpringStiffnessUnits=m*N/rad  DampingCoefficient=0  DampingCoefficientUnits=m*s*N/rad  TorqueActuationMode=NoTorque  MotionActuationMode=ComputedMotion  SensePosition=off  SenseVelocity=off  SenseAcceleration=off  SenseTorqueForce=off  SenseLowerLimitTorqueForce=off  SenseUpperLimitTorqueForce=off  LowerLimitSpecify=off  LowerLimitBound=-90  LowerLimitBoundUnits=deg  LowerLimitStiffness=1e4  LowerLimitStiffnessUnits=N*m/deg  LowerLimitDamping=10  LowerLimitDampingUnits=N*m/(deg/s)  LowerLimitTransitionRegionWidth=0.1  LowerLimitTransitionRegionWidthUnits=deg  UpperLimitSpecify=off  UpperLimitBound=90  UpperLimitBoundUnits=deg  UpperLimitStiffness=1e4  UpperLimitStiffnessUnits=N*m/deg  UpperLimitDamping=10  UpperLimitDampingUnits=N*m/(deg/s)  UpperLimitTransitionRegionWidth=0.1  UpperLimitTransitionRegionWidthUnits=deg  PositionTargetSpecify=on  PositionTargetPriority=High  PositionTargetValue=-90  PositionTargetValueUnits=deg  VelocityTargetSpecify=on  VelocityTargetPriority=High  VelocityTargetValue=0  VelocityTargetValueUnits=deg/s
  Solver Configuration : nesl_utility/Solver Configuration  PhysicalDomain=network_engine_domain  SubClassName=solver  LeftPortType=input  RightPortType=generic  Tones=[]  Harmonics=[]  SimulateNoise=off  Profile=off  UseLocalSampling=off  EnableSwitchedLinearOptims=on  FrequencyDomain=off  UseCCode=off  RelTol=0.001  AbsTol=1e-06  MinStep=1e-09  ToWorkspace=off  RevertToSquareIcSolve=off  NumHomotopyIterations=100  PhasorMode=off  PhasorModeNumHarmonics=1  DoDC=off  ResidualTolerance=1e-09  UseLocalSolver=off  LocalSolverChoice=NE_BACKWARD_EULER_ADVANCER  LocalSolverSampleTime=0.001  DoFixedCost=off  MaxNonlinIter=3  MaxModeIter=2  LinearAlgebra=Sparse  EquationFormulation=NE_TIME_EF  DelaysMemoryBudget=1024  AutomaticFiltering=on  FilteringTimeConstant=0.001  PartitionStorageMethod=AS_NEEDED  PartitionMemoryBudget=1024  PartitionMethod=FAST
      settings: SourceProductBaseCode=MT,SS
  Transforn : sm_lib/Frames and Transforms/Rigid Transform  TranslationMethod=None  TranslationStandardOffset=0  TranslationLengthUnit=m  TranslationStandardAxis=+Z  TranslationCartesianOffset=[0 0 0]  TranslationROffset=0  TranslationROffsetUnits=m  TranslationZOffset=0  TranslationZOffsetUnits=m  TranslationThetaOffset=0  TranslationThetaOffsetUnits=deg  RotationMethod=None  RotationAngleUnits=deg  RotationStandardAxis=+Z  RotationAngle=0.0  RotationArbitraryAxis=[0 0 1]  FollAlignAxisA=+X  BaseAlignAxisA=+Y  FollAlignAxisB=+Y  BaseAlignAxisB=+Z  RotationSequenceAxes=FollowerAxes  RotationSequence=XYX  RotationSequenceAngles=[0 0 0]  RotationSequenceAnglesUnits=deg  RotationMatrix=[1 0 0; 0 1 0; 0 0 1]
  Turntable : Subsystem
      mask Display: image('Turntable.jpg')
  World : sm_lib/Frames and Transforms/World Frame
  Wrist : Subsystem
      mask Display: image('Wrist.jpg')
  tTin : PMIOPort  Side=Left
  tA : PMIOPort  Port=2  Side=Right
  tW : PMIOPort  Port=3  Side=Left
  bTin : PMIOPort  Port=4  Side=Left
  bA : PMIOPort  Port=5  Side=Right
  bW : PMIOPort  Port=6  Side=Left
  fTin : PMIOPort  Port=7  Side=Left
  fA : PMIOPort  Port=8  Side=Right
  fW : PMIOPort  Port=9  Side=Left
  wTin : PMIOPort  Port=10  Side=Left
  wA : PMIOPort  Port=11  Side=Right
  wW : PMIOPort  Port=12  Side=Left
  hTin : PMIOPort  Port=13  Side=Left
  hA : PMIOPort  Port=14  Side=Right
  hW : PMIOPort  Port=15  Side=Left
  gTin : PMIOPort  Port=16  Side=Left
  gA : PMIOPort  Port=17  Side=Right
  gW : PMIOPort  Port=18  Side=Left
  connections:
  World/RConn1 -- Transforn/LConn1 -- MechanismConfiguration/RConn1 -- Solver Configuration/RConn1
  R2/LConn1 -- Turntable/RConn2
  Gripper/LConn3 -- R7/RConn1
  Hand/RConn2 -- P2/LConn1
  Gripper/LConn2 -- P2/RConn1
  R6/LConn1 -- Wrist/RConn1
  Hand/LConn2 -- R6/RConn1
  Hand/RConn1 -- P1/LConn1
  Gripper/LConn1 -- P1/RConn1
  Forearm/RConn1 -- R4/LConn1
  R4/RConn1 -- Wrist/LConn1
  Base/LConn1 -- Transforn/RConn1
  Bicep/LConn1 -- R2/RConn1
  Bicep/RConn1 -- R3/LConn1
  Forearm/LConn2 -- R3/RConn1
  R5/LConn1 -- Wrist/RConn2
  DriveGear/LConn2 -- R5/RConn1
  Base/RConn1 -- R1/LConn1
  R1/RConn1 -- Turntable/LConn1
  Hand/RConn3 -- R7/LConn1
  tTin/RConn1 -- R1/LConn2
  bTin/RConn1 -- R2/LConn2
  fTin/RConn1 -- R3/LConn2
  wTin/RConn1 -- R4/LConn2
  hTin/RConn1 -- R5/LConn2
  gTin/RConn1 -- R7/LConn2
  Gear Constraint/LConn1 -- DriveGear/LConn1
  Gear Constraint/RConn1 -- Hand/LConn3
  R1/RConn2 -- tA/RConn1
  R1/RConn3 -- tW/RConn1
  R2/RConn2 -- bA/RConn1
  R2/RConn3 -- bW/RConn1
  R3/RConn2 -- fA/RConn1
  R3/RConn3 -- fW/RConn1
  R4/RConn2 -- wA/RConn1
  R4/RConn3 -- wW/RConn1
  R5/RConn2 -- hA/RConn1
  R5/RConn3 -- hW/RConn1
  R7/RConn2 -- gA/RConn1
  R7/RConn3 -- gW/RConn1

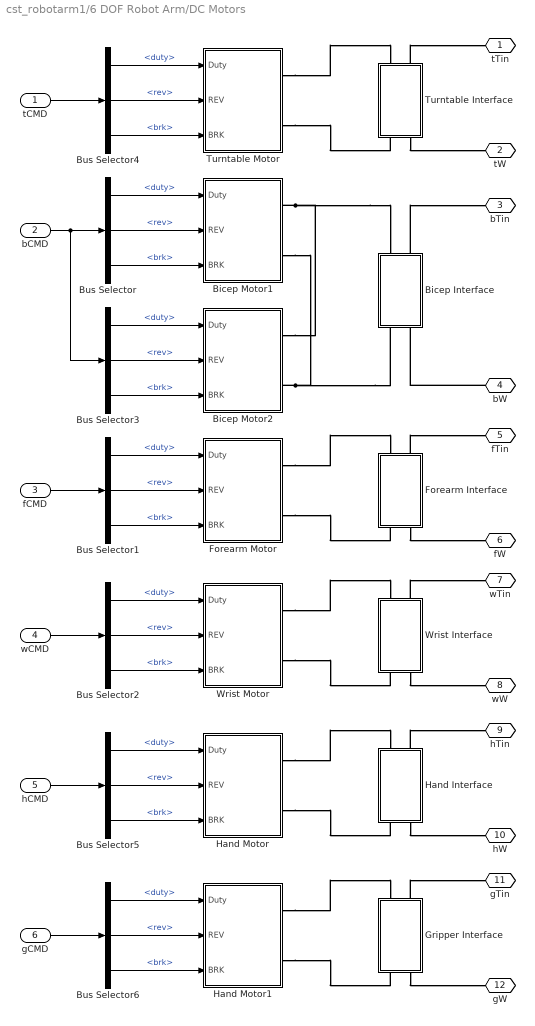
== system cst_robotarm1/6 DOF Robot Arm/DC Motors ==
  tCMD : Inport
  bCMD : Inport  Port=2
  fCMD : Inport  Port=3
  wCMD : Inport  Port=4
  hCMD : Inport  Port=5
  gCMD : Inport  Port=6
  Bicep Interface : Subsystem
  Bicep Motor1 : Subsystem
      mask Display: image('Servo.jpg')
  Bicep Motor2 : Subsystem
      mask Display: image('Servo.jpg')
  Bus Selector{,1..6} (7 alike) : BusSelector  OutputSignals=duty,rev,brk
  Forearm Interface : Subsystem
  Forearm Motor : Subsystem
      mask Display: image('Servo.jpg')
  Gripper Interface : Subsystem
  Hand Interface : Subsystem
  Hand Motor : Subsystem
      mask Display: image('Servo.jpg')
  Hand Motor1 : Subsystem
      mask Display: image('Servo.jpg')
  Turntable Interface : Subsystem
  Turntable Motor : Subsystem
      mask Display: image('Servo.jpg')
  Wrist Interface : Subsystem
  Wrist Motor : Subsystem
      mask Display: image('Servo.jpg')
  tTin : PMIOPort  Side=Right
  tW : PMIOPort  Port=2  Side=Right
  bTin : PMIOPort  Port=3  Side=Right
  bW : PMIOPort  Port=4  Side=Right
  fTin : PMIOPort  Port=5  Side=Right
  fW : PMIOPort  Port=6  Side=Right
  wTin : PMIOPort  Port=7  Side=Right
  wW : PMIOPort  Port=8  Side=Right
  hTin : PMIOPort  Port=9  Side=Right
  hW : PMIOPort  Port=10  Side=Right
  gTin : PMIOPort  Port=11  Side=Right
  gW : PMIOPort  Port=12  Side=Right
  wires:
  bCMD/1 -> Bus Selector/1, Bus Selector3/1
  Bus Selector/1 -> Bicep Motor1/1(Duty)  "<duty>"
  Bus Selector/2 -> Bicep Motor1/2(REV)  "<rev>"
  Bus Selector/3 -> Bicep Motor1/3(BRK)  "<brk>"
  fCMD/1 -> Bus Selector1/1
  Bus Selector1/1 -> Forearm Motor/1(Duty)  "<duty>"
  Bus Selector1/2 -> Forearm Motor/2(REV)  "<rev>"
  Bus Selector1/3 -> Forearm Motor/3(BRK)  "<brk>"
  Bus Selector3/1 -> Bicep Motor2/1(Duty)  "<duty>"
  Bus Selector3/2 -> Bicep Motor2/2(REV)  "<rev>"
  Bus Selector3/3 -> Bicep Motor2/3(BRK)  "<brk>"
  wCMD/1 -> Bus Selector2/1
  Bus Selector2/1 -> Wrist Motor/1(Duty)  "<duty>"
  Bus Selector2/2 -> Wrist Motor/2(REV)  "<rev>"
  Bus Selector2/3 -> Wrist Motor/3(BRK)  "<brk>"
  tCMD/1 -> Bus Selector4/1
  Bus Selector4/1 -> Turntable Motor/1(Duty)  "<duty>"
  Bus Selector4/2 -> Turntable Motor/2(REV)  "<rev>"
  Bus Selector4/3 -> Turntable Motor/3(BRK)  "<brk>"
  hCMD/1 -> Bus Selector5/1
  Bus Selector5/1 -> Hand Motor/1(Duty)  "<duty>"
  Bus Selector5/2 -> Hand Motor/2(REV)  "<rev>"
  Bus Selector5/3 -> Hand Motor/3(BRK)  "<brk>"
  gCMD/1 -> Bus Selector6/1
  Bus Selector6/1 -> Hand Motor1/1(Duty)  "<duty>"
  Bus Selector6/2 -> Hand Motor1/2(REV)  "<rev>"
  Bus Selector6/3 -> Hand Motor1/3(BRK)  "<brk>"
  connections:
  Bicep Motor1/RConn1 -- Bicep Motor2/RConn1 -- Bicep Interface/LConn1
  Bicep Motor2/RConn2 -- Bicep Motor1/RConn2 -- Bicep Interface/RConn1
  Forearm Motor/RConn2 -- Forearm Interface/RConn1
  Forearm Motor/RConn1 -- Forearm Interface/LConn1
  Forearm Interface/RConn2 -- fW/RConn1
  Bicep Interface/LConn2 -- bTin/RConn1
  Forearm Interface/LConn2 -- fTin/RConn1
  bW/RConn1 -- Bicep Interface/RConn2
  Wrist Motor/RConn2 -- Wrist Interface/RConn1
  Wrist Interface/LConn2 -- wTin/RConn1
  Wrist Motor/RConn1 -- Wrist Interface/LConn1
  Wrist Interface/RConn2 -- wW/RConn1
  Turntable Interface/LConn2 -- tTin/RConn1
  Turntable Motor/RConn1 -- Turntable Interface/LConn1
  Turntable Motor/RConn2 -- Turntable Interface/RConn1
  Turntable Interface/RConn2 -- tW/RConn1
  Hand Interface/RConn2 -- hW/RConn1
  Hand Motor/RConn1 -- Hand Interface/LConn1
  Hand Interface/LConn2 -- hTin/RConn1
  Hand Motor/RConn2 -- Hand Interface/RConn1
  Hand Motor1/RConn2 -- Gripper Interface/RConn1
  Gripper Interface/RConn2 -- gW/RConn1
  Hand Motor1/RConn1 -- Gripper Interface/LConn1
  Gripper Interface/LConn2 -- gTin/RConn1
